simulink model "OFDM_Simulation_QPSK_rs1"  (R2018b)
settings: Solver=ode45  StartTime=0.0  StopTime=0.08  RelTol=1e-3  EnableMultiTasking=on
undefined symbols (not defined in the file or in its folder): doppler, rsgenpoly
libraries: dspindex x4, commdigbbndpm3 x4, commchan3 x2, commblkcod2 x2, commseqgen2 x2, commutil2 x2, dspxfrm3 x2, commrandsrc2 x1, commsink2 x1, dspobslib x1, dspsigops x1
settings Model: Creator=Three  LastModifiedBy=18831
settings SolverCC: MaxConsecutiveZCs=10
settings DataIOCC: LimitDataPoints=on  SaveFormat=Array
settings OptimizationCC: LifeSpan=inf
settings DebuggingCC: SolverPrmCheckMsg=warning  SFUnexpectedBacktrackingDiag=warning  SFNoUnconditionalDefaultTransitionDiag=warning  SFExecutionAtInitializationDiag=none
settings HardwareCC: ProdBitPerPointer=32  ProdBitPerSizeT=32  ProdBitPerPtrDiffT=32  ProdLargestAtomicFloat=None  ProdIntDivRoundTo=Undefined  ProdEndianess=Unspecified  ProdWordSize=32  ProdHWDeviceType=32-bit Generic
settings ModelReferenceCC: PropagateSignalLabelsOutOfModel=off
settings SFSimCC: SimUseLocalCustomCode=off
settings RTWCC: RTWUseLocalCustomCode=off
settings CodeAppCC: StateflowObjectComments=on
settings GRTTargetCC: TargetLangStandard=C89/C90 (ANSI)  GeneratePreprocessorConditionals=Disable all
settings ConfigComp: CovMetricSettings=dw  CovHtmlReporting=on  CovSaveCumulativeToWorkspaceVar=on  CovSaveSingleToWorkspaceVar=on  CovExternalEMLEnable=off  CovSFcnEnable=off

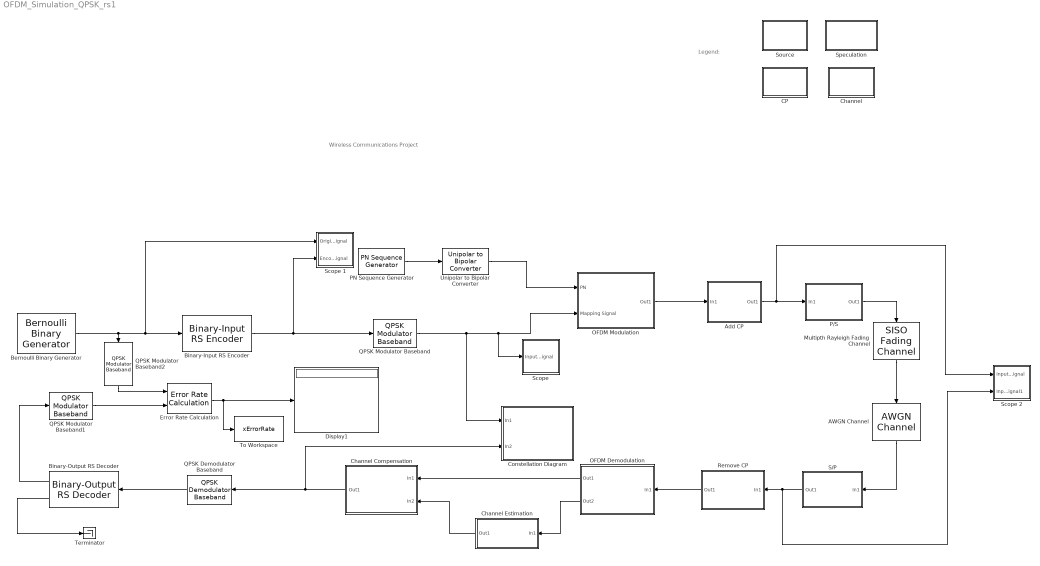
== system OFDM_Simulation_QPSK_rs1 ==
  note: Legend:
  note: Wireless Communications Project
  " Add CP" : Subsystem  TreatAsAtomicUnit=on
      mask Display: disp('Add CP')
  AWGN Channel : commchan3/AWGN Channel  InputProcessing=Columns as channels (frame based)  seed=17  noiseMode="Signal to noise ratio  (SNR)"  EbNodB=10  EsNodB=10  SNRdB=20  bitsPerSym=1  Ps=0.007  Tsym=1  variance=1
  Bernoulli Binary Generator : commrandsrc2/Bernoulli Binary Generator  P=0.5  seed=9044  Ts=16e-5/88/2  frameBased=on  sampPerFrame=88  orient=off  outDataType=double
  Binary-Input RS Encoder : commblkcod2/Binary-Input RS Encoder  n=15  k=11  specShortening=off  shortenedK=3  specGenPoly=off  genPoly=rsgenpoly(7,3)  specPrimPoly=off  prPoly=[1 0 1 1]  specPuncture=off  punctVec=[ones(2,1); zeros(2,1)]  outDType=Same as input
      settings: SourceProductName=Communications System Toolbox  SourceProductBaseCode=CM
  Binary-Output RS Decoder : commblkcod2/Binary-Output RS Decoder  n=15  k=11  specShortening=off  shortenedK=3  specGenPoly=off  genPoly=rsgenpoly(7,3)  specPrimPoly=off  prPoly=[1 0 1 1]  specPuncture=off  punctVec=[ones(2,1); zeros(2,1)]  specErasurePort=off  showNumErr=on  outDType=Same as input
      settings: SourceProductName=Communications System Toolbox  SourceProductBaseCode=CM
  CP : Subsystem  TreatAsAtomicUnit=on
      mask Display: disp('CP')
  Channel : Subsystem  TreatAsAtomicUnit=on
      mask Display: disp('Channel')
  Channel Compensation : Subsystem  TreatAsAtomicUnit=on
      mask Display: disp('Channel Compensation')
  Channel Estimation : Subsystem  TreatAsAtomicUnit=on
      mask Display: disp('Channel Estimation')
  Constellation Diagram : Subsystem  TreatAsAtomicUnit=on
      mask Display: disp('Constellation Diagram')
  Display1 : Display
  Error Rate Calculation : commsink2/Error Rate Calculation  N=44  st_delay=0  cp_mode=Entire frame  subframe=[]  PMode=Port  WsName=xErrorRate  RsMode2=off  stop=off  numErr=100  maxBits=1e6
  Multipth Rayleigh Fading Channel : commchan3/SISO Fading Channel  InheritSampleRate=on  SampleRate=1  PathDelays=[0 2e-6]  AveragePathGains=[0 -3]  NormalizePathGains=on  FadingDistribution=Rayleigh  KFactor=3  DirectPathDopplerShift=0  DirectPathInitialPhase=0  MaximumDopplerShift=100  DopplerSpectrum=doppler('Jakes')  ChannelInterpolationMethod=Polyphase  RandomStream=mt19937ar with seed  RandomNumGenerator=shr3cong  Seed=8007  PathGainsOutputPort=off  ChannelFilterDelayOutputPort=off  SimulateUsing=Interpreted execution  Visualization=Off  PathsForDopplerDisplay=1  SamplesToDisplay=25%
      settings: SourceProductName=Communications System Toolbox
  OFDM Demodulation : Subsystem  TreatAsAtomicUnit=on
      mask Display: disp('OFDM Demodulation')
  OFDM Modulation : Subsystem  TreatAsAtomicUnit=on
      mask Display: disp('OFDM Modulation')
  P/S : Subsystem  TreatAsAtomicUnit=on
      mask Display: disp('P/S')
  PN Sequence Generator : commseqgen2/PN Sequence Generator  poly=[1 0 0 0 0 1 1]  ini_sta=[0 0 0 0 0 1]  outBitMaskSource=Dialog parameter  shift=0  outVarSiz=off  maxOutSizeMode=Dialog parameter  maxOutSize=[10 1]  Ts=16e-5/2/61  frameBased=on  sampPerFrame=61  reset=off  bitPackedOutputs=off  outDataType=double  numPackedBits=8  bitPackDataSigned=off  bitPackedOutDType=double
  QPSK Demodulator Baseband : commdigbbndpm3/QPSK Demodulator Baseband  OutType=Bit  DecType=Hard decision  VarSource=Dialog  Variance=1  Dec=Gray  Ph=pi/4  outDtype1=Inherit via internal rule  outDtype2=Inherit via internal rule  derotateFactorWordLen=16  derotateFactorDataTypeStr=Inherit: Same word length as input  derotateFactorLastDataTypeStr=Inherit: Same word length as input
  QPSK Modulator Baseband : commdigbbndpm3/QPSK Modulator Baseband  InType=Bit  Enc=Gray  Ph=pi/4  outDtype=double  outWordLen=16  outUDDataType=sfix(16)  outFracLenMode=Best precision  outFracLen=15  outDataTypeStr=double  outLastDataTypeStr=double
  QPSK Modulator Baseband1 : commdigbbndpm3/QPSK Modulator Baseband  InType=Bit  Enc=Binary  Ph=pi/4  outDtype=double  outWordLen=16  outUDDataType=sfix(16)  outFracLenMode=Best precision  outFracLen=15  outDataTypeStr=double  outLastDataTypeStr=double
  QPSK Modulator Baseband2 : commdigbbndpm3/QPSK Modulator Baseband  InType=Bit  Enc=Binary  Ph=pi/4  outDtype=double  outWordLen=16  outUDDataType=sfix(16)  outFracLenMode=Best precision  outFracLen=15  outDataTypeStr=double  outLastDataTypeStr=double
  Remove CP : Subsystem  TreatAsAtomicUnit=on
      mask Display: disp('Remove CP')
  S/P : Subsystem  TreatAsAtomicUnit=on
      mask Display: disp('S/P')
  "Scope " : Subsystem
      mask Display: disp('Scope')
  Scope 1 : Subsystem
      mask Display: disp('Scope')
  Scope 2 : Subsystem
      mask Display: disp('Scope')
  Source : Subsystem  TreatAsAtomicUnit=on
      mask Display: disp('Source')
  Speculation : Subsystem  TreatAsAtomicUnit=on
      mask Display: disp('Speculation')
  Terminator : Terminator
  To Workspace : ToWorkspace  VariableName=xErrorRate  SampleTime=-1
      settings: Save2DSignal=2-D array (concatenate along first dimension)
  Unipolar to Bipolar Converter : commutil2/Unipolar to Bipolar Converter  M=2  polarity=Positive  dataType=Inherit via internal rule
      settings: SourceProductName=Communications System Toolbox
  wires:
  PN Sequence Generator/1 -> Unipolar to Bipolar Converter/1
  Unipolar to Bipolar Converter/1 -> OFDM Modulation/1(PN)
  QPSK Modulator Baseband/1 -> "Scope "/1(Input Signal), OFDM Modulation/2(Mapping Signal), Constellation Diagram/1(In1)
  Bernoulli Binary Generator/1 -> QPSK Modulator Baseband2/1, Scope 1/1(Original Signal), Binary-Input RS Encoder/1
  OFDM Modulation/1(Out1) -> " Add CP"/1(In1)
  " Add CP"/1(Out1) -> Scope 2/1(Input Signal), P/S/1(In1)
  AWGN Channel/1 -> S/P/1(In1)
  Remove CP/1(Out1) -> OFDM Demodulation/1(In1)
  OFDM Demodulation/2(Out2) -> Channel Estimation/1(In1)
  Channel Estimation/1(Out1) -> Channel Compensation/2(In2)
  OFDM Demodulation/1(Out1) -> Channel Compensation/1(In1)
  Channel Compensation/1(Out1) -> Constellation Diagram/2(In2), QPSK Demodulator Baseband/1
  QPSK Modulator Baseband1/1 -> Error Rate Calculation/2
  QPSK Modulator Baseband2/1 -> Error Rate Calculation/1
  P/S/1(Out1) -> Multipth Rayleigh Fading Channel/1
  Multipth Rayleigh Fading Channel/1 -> AWGN Channel/1
  Binary-Output RS Decoder/2 -> Terminator/1
  Binary-Input RS Encoder/1 -> QPSK Modulator Baseband/1, Scope 1/2(Encoded Signal)
  Error Rate Calculation/1 -> To Workspace/1, Display1/1
  QPSK Demodulator Baseband/1 -> Binary-Output RS Decoder/1
  Binary-Output RS Decoder/1 -> QPSK Modulator Baseband1/1
  S/P/1(Out1) -> Scope 2/2(Input Signal1), Remove CP/1(In1)

== system OFDM_Simulation_QPSK_rs1/ Add CP ==
  In1 : Inport
  Selector : Selector  NumberOfDimensions=2  InputPortWidth=3  IndexOptions=Index vector (dialog),Select all  Indices=[39:64,1:64],1  OutputSizes=1,1
  Out1 : Outport
  wires:
  In1/1 -> Selector/1
  Selector/1 -> Out1/1

== system OFDM_Simulation_QPSK_rs1/CP ==

== system OFDM_Simulation_QPSK_rs1/Channel ==

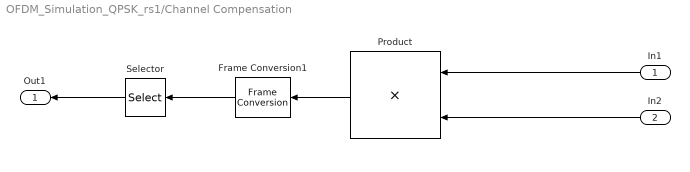
== system OFDM_Simulation_QPSK_rs1/Channel Compensation ==
  In1 : Inport
  In2 : Inport  Port=2
  Frame Conversion1 : FrameConversion
  Product : Product
  Selector : Selector  NumberOfDimensions=2  InputPortWidth=3  IndexOptions=Index vector (dialog),Select all  Indices=[1:30,32:61],1  OutputSizes=1,1
  Out1 : Outport
  wires:
  In1/1 -> Product/1
  In2/1 -> Product/2
  Product/1 -> Frame Conversion1/1
  Frame Conversion1/1 -> Selector/1
  Selector/1 -> Out1/1

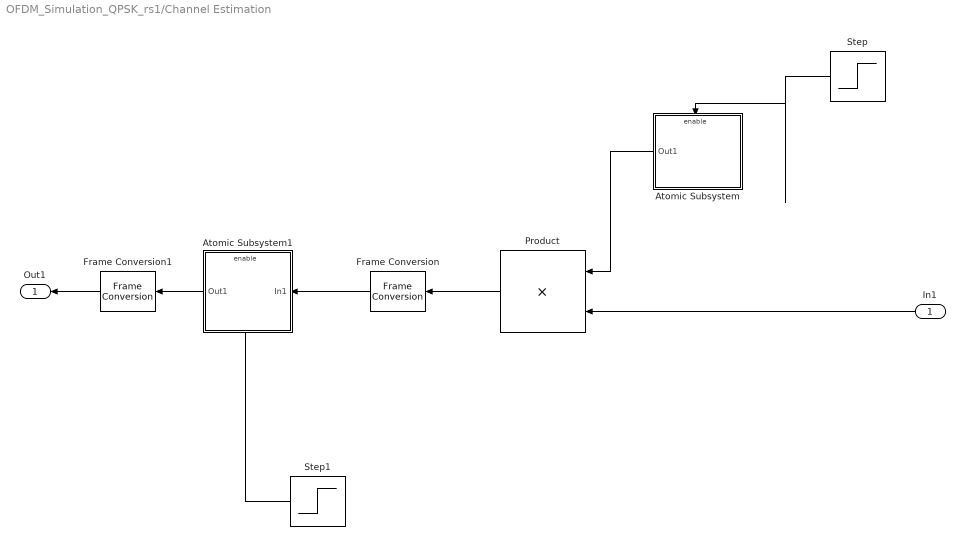
== system OFDM_Simulation_QPSK_rs1/Channel Estimation ==
  In1 : Inport
  Atomic Subsystem : Subsystem  TreatAsAtomicUnit=on
  Atomic Subsystem1 : Subsystem  TreatAsAtomicUnit=on
  Frame Conversion : FrameConversion
  Frame Conversion1 : FrameConversion
  Product : Product
  Step : Step  Time=16e-5/2  SampleTime=0
  Step1 : Step  Time=16e-5/2  SampleTime=0
  Out1 : Outport
  wires:
  In1/1 -> Product/2
  Step/1 -> Atomic Subsystem/Enable
  Atomic Subsystem/1(Out1) -> Product/1
  Product/1 -> Frame Conversion/1
  Frame Conversion/1 -> Atomic Subsystem1/1(In1)
  Step1/1 -> Atomic Subsystem1/Enable
  Atomic Subsystem1/1(Out1) -> Frame Conversion1/1
  Frame Conversion1/1 -> Out1/1

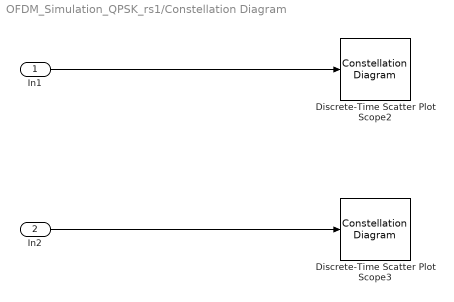
== system OFDM_Simulation_QPSK_rs1/Constellation Diagram ==
  In1 : Inport
  In2 : Inport  Port=2
  Discrete-Time Scatter Plot Scope2 : ConstellationDiagram  Tag=ScatterPlot
  Discrete-Time Scatter Plot Scope3 : ConstellationDiagram  Tag=ScatterPlot
  wires:
  In2/1 -> Discrete-Time Scatter Plot Scope3/1
  In1/1 -> Discrete-Time Scatter Plot Scope2/1

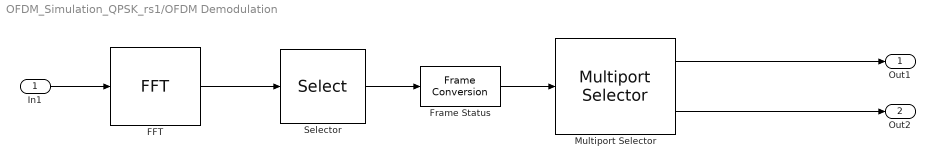
== system OFDM_Simulation_QPSK_rs1/OFDM Demodulation ==
  In1 : Inport
  FFT : dspxfrm3/FFT  FFTImplementation=Auto  CompMethod=Table lookup  TableOpt=NEW  TableOptActive=Speed  BitRevOrder=off  Normalize=off  InheritFFTLength=on  FFTLength=64  WrapInput=on  roundingMode=Floor  overflowMode=off  firstCoeffDataTypeStr=Inherit: Same word length as input  firstCoeffLastDataTypeStr=Inherit: Same word length as input  outputMin=[]  outputMax=[]
  Frame Status : FrameConversion
  Multiport Selector : dspindex/Multiport Selector  rowsOrCols=Columns  idxCellArray={1,2}  idxErrMode=Clip Index
  Selector : Selector  NumberOfDimensions=2  InputPortWidth=3  IndexOptions=Index vector (dialog),Select all  Indices=[35:64,1:31],1  OutputSizes=1,1
  Out1 : Outport
  Out2 : Outport  Port=2
  wires:
  In1/1 -> FFT/1
  FFT/1 -> Selector/1
  Selector/1 -> Frame Status/1
  Frame Status/1 -> Multiport Selector/1
  Multiport Selector/2 -> Out2/1
  Multiport Selector/1 -> Out1/1

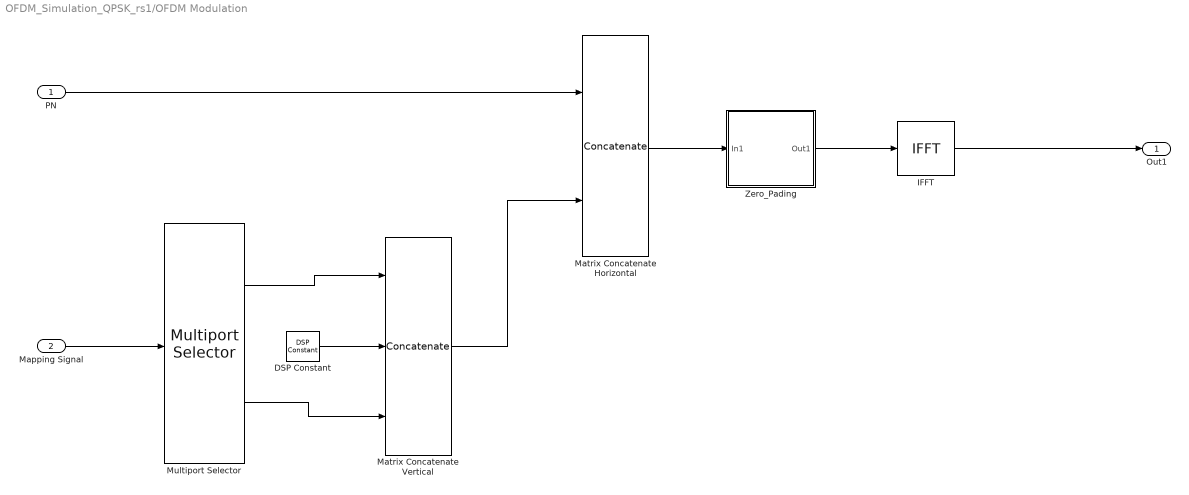
== system OFDM_Simulation_QPSK_rs1/OFDM Modulation ==
  PN : Inport
  Mapping Signal : Inport  Port=2
  DSP Constant : dspobslib/DSP Constant  Value=0  SampleMode=Discrete  discreteOutput=Frame-based  continuousOutput=Sample-based  sampTime=16e-5/2  framePeriod=16e-5/2  dataType=Inherit from 'Constant value'  isSigned=on  wordLen=16  udDataType=sfix(16)  fracBitsMode=Best precision  numFracBits=15  InterpretAs1D=off  Ts=16e-5/2  FramebasedOutput=on
      settings: SourceProductName=DSP System Toolbox  SourceProductBaseCode=DS
  IFFT : dspxfrm3/IFFT  FFTImplementation=Auto  CompMethod=Table lookup  TableOpt=NEW  TableOptActive=Speed  BitRevOrder=off  cs_in=off  Normalize=on  InheritFFTLength=on  FFTLength=64  WrapInput=on  mode=Complex  outSamplingMode=Frame based  roundingMode=Floor  overflowMode=off  firstCoeffDataTypeStr=Inherit: Same word length as input  firstCoeffLastDataTypeStr=Inherit: Same word length as input  outputMin=[]  outputMax=[]
      settings: SourceProductName=DSP System Toolbox
  Matrix Concatenate Horizontal : Concatenate  Mode=Multidimensional array  ConcatenateDimension=2
  Matrix Concatenate Vertical : Concatenate  NumInputs=3  Mode=Multidimensional array
  Multiport Selector : dspindex/Multiport Selector  rowsOrCols=Rows  idxCellArray={1:30,31:60}  idxErrMode=Clip Index
  Zero_Pading : Subsystem  TreatAsAtomicUnit=on
      mask Display: disp('Zero_Pading')
  Out1 : Outport
  wires:
  Mapping Signal/1 -> Multiport Selector/1
  PN/1 -> Matrix Concatenate Horizontal/1
  Multiport Selector/1 -> Matrix Concatenate Vertical/1
  Multiport Selector/2 -> Matrix Concatenate Vertical/3
  DSP Constant/1 -> Matrix Concatenate Vertical/2
  Matrix Concatenate Vertical/1 -> Matrix Concatenate Horizontal/2
  Matrix Concatenate Horizontal/1 -> Zero_Pading/1(In1)
  Zero_Pading/1(Out1) -> IFFT/1
  IFFT/1 -> Out1/1

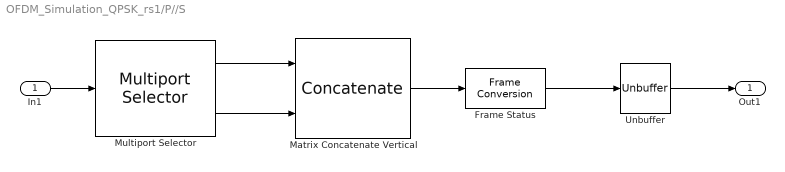
== system OFDM_Simulation_QPSK_rs1/P//S ==
  In1 : Inport
  Frame Status : FrameConversion
  Matrix Concatenate Vertical : Concatenate  Mode=Multidimensional array
  Multiport Selector : dspindex/Multiport Selector  rowsOrCols=Columns  idxCellArray={1,2}  idxErrMode=Clip Index
  Unbuffer : Unbuffer
  Out1 : Outport
  wires:
  In1/1 -> Multiport Selector/1
  Multiport Selector/1 -> Matrix Concatenate Vertical/1
  Multiport Selector/2 -> Matrix Concatenate Vertical/2
  Matrix Concatenate Vertical/1 -> Frame Status/1
  Frame Status/1 -> Unbuffer/1
  Unbuffer/1 -> Out1/1

== system OFDM_Simulation_QPSK_rs1/Remove CP ==
  In1 : Inport
  Selector : Selector  NumberOfDimensions=2  InputPortWidth=3  IndexOptions=Index vector (dialog),Select all  Indices=[27:90],1  OutputSizes=1,1
  Out1 : Outport
  wires:
  In1/1 -> Selector/1
  Selector/1 -> Out1/1

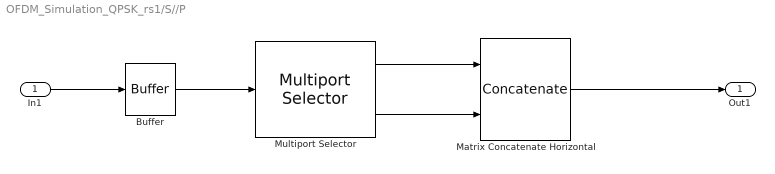
== system OFDM_Simulation_QPSK_rs1/S//P ==
  In1 : Inport
  Buffer : Buffer  N=180
  Matrix Concatenate Horizontal : Concatenate  Mode=Multidimensional array  ConcatenateDimension=2
  Multiport Selector : dspindex/Multiport Selector  rowsOrCols=Rows  idxCellArray={91:180,1:90}  idxErrMode=Clip Index
  Out1 : Outport
  wires:
  In1/1 -> Buffer/1
  Buffer/1 -> Multiport Selector/1
  Multiport Selector/1 -> Matrix Concatenate Horizontal/1
  Multiport Selector/2 -> Matrix Concatenate Horizontal/2
  Matrix Concatenate Horizontal/1 -> Out1/1

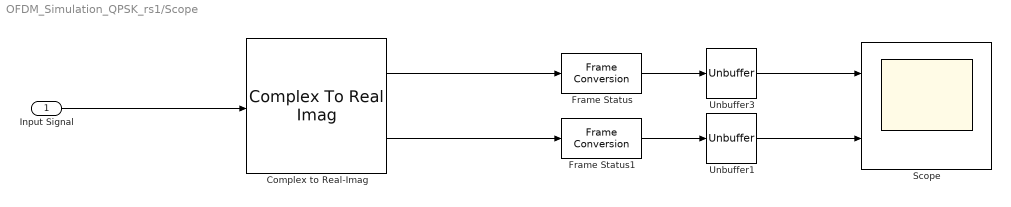
== system OFDM_Simulation_QPSK_rs1/Scope  ==
  Input Signal : Inport
  Complex to Real-Imag : ComplexToRealImag
  Frame Status : FrameConversion  OutFrame=Sample-based
  Frame Status1 : FrameConversion  OutFrame=Sample-based
  Scope : Scope  NumInputPorts=2
  Unbuffer1 : Unbuffer
  Unbuffer3 : Unbuffer
  wires:
  Input Signal/1 -> Complex to Real-Imag/1
  Complex to Real-Imag/2 -> Frame Status1/1
  Frame Status1/1 -> Unbuffer1/1
  Unbuffer1/1 -> Scope/2
  Unbuffer3/1 -> Scope/1
  Complex to Real-Imag/1 -> Frame Status/1
  Frame Status/1 -> Unbuffer3/1

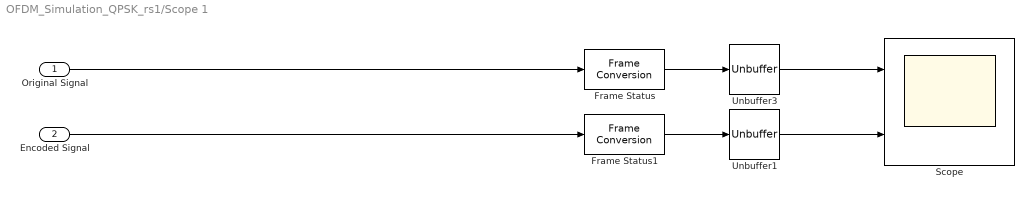
== system OFDM_Simulation_QPSK_rs1/Scope 1 ==
  Original Signal : Inport
  Encoded Signal : Inport  Port=2
  Frame Status : FrameConversion  OutFrame=Sample-based
  Frame Status1 : FrameConversion  OutFrame=Sample-based
  Scope : Scope  NumInputPorts=2
  Unbuffer1 : Unbuffer
  Unbuffer3 : Unbuffer
  wires:
  Frame Status1/1 -> Unbuffer1/1
  Unbuffer1/1 -> Scope/2
  Unbuffer3/1 -> Scope/1
  Frame Status/1 -> Unbuffer3/1
  Encoded Signal/1 -> Frame Status1/1
  Original Signal/1 -> Frame Status/1

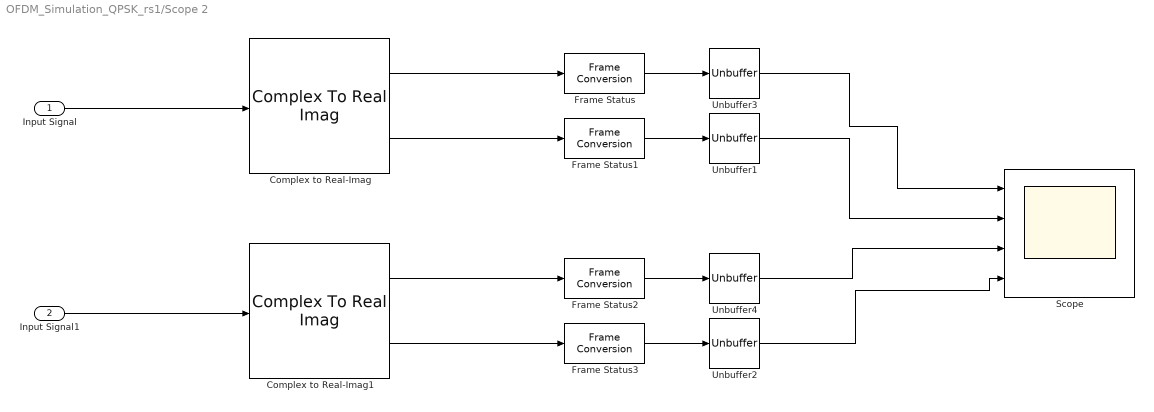
== system OFDM_Simulation_QPSK_rs1/Scope 2 ==
  Input Signal : Inport
  Input Signal1 : Inport  Port=2
  Complex to Real-Imag : ComplexToRealImag
  Complex to Real-Imag1 : ComplexToRealImag
  Frame Status{,1..3} (4 alike) : FrameConversion  OutFrame=Sample-based
  Scope : Scope  NumInputPorts=4
  Unbuffer{1..4} (4 alike) : Unbuffer
  wires:
  Input Signal/1 -> Complex to Real-Imag/1
  Complex to Real-Imag/2 -> Frame Status1/1
  Frame Status1/1 -> Unbuffer1/1
  Unbuffer1/1 -> Scope/2
  Unbuffer3/1 -> Scope/1
  Complex to Real-Imag/1 -> Frame Status/1
  Frame Status/1 -> Unbuffer3/1
  Input Signal1/1 -> Complex to Real-Imag1/1
  Complex to Real-Imag1/2 -> Frame Status3/1
  Frame Status3/1 -> Unbuffer2/1
  Unbuffer2/1 -> Scope/4
  Unbuffer4/1 -> Scope/3
  Complex to Real-Imag1/1 -> Frame Status2/1
  Frame Status2/1 -> Unbuffer4/1

== system OFDM_Simulation_QPSK_rs1/Source ==

== system OFDM_Simulation_QPSK_rs1/Speculation ==

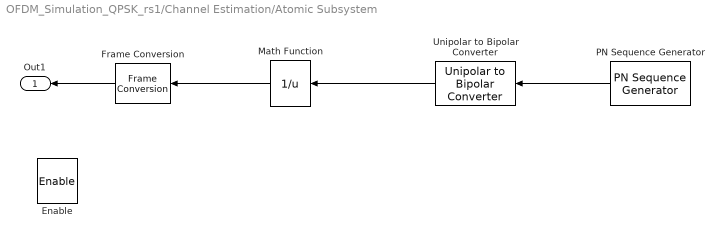
== system OFDM_Simulation_QPSK_rs1/Channel Estimation/Atomic Subsystem ==
  Enable : EnablePort
  Frame Conversion : FrameConversion
  Math Function : Math  Operator=reciprocal  SaturateOnIntegerOverflow=on
  PN Sequence Generator : commseqgen2/PN Sequence Generator  poly=[1 0 0 0 0 1 1]  ini_sta=[0 0 0 0 0 1]  outBitMaskSource=Dialog parameter  shift=0  outVarSiz=off  maxOutSizeMode=Dialog parameter  maxOutSize=[10 1]  Ts=16e-5/2/61  frameBased=on  sampPerFrame=61  reset=off  bitPackedOutputs=off  outDataType=double  numPackedBits=8  bitPackDataSigned=off  bitPackedOutDType=double
  Unipolar to Bipolar Converter : commutil2/Unipolar to Bipolar Converter  M=2  polarity=Positive  dataType=Inherit via internal rule
      settings: SourceProductName=Communications System Toolbox
  Out1 : Outport
  wires:
  PN Sequence Generator/1 -> Unipolar to Bipolar Converter/1
  Frame Conversion/1 -> Out1/1
  Unipolar to Bipolar Converter/1 -> Math Function/1
  Math Function/1 -> Frame Conversion/1

== system OFDM_Simulation_QPSK_rs1/Channel Estimation/Atomic Subsystem1 ==
  In1 : Inport
  Enable : EnablePort
  Math Function : Math  Operator=reciprocal  SaturateOnIntegerOverflow=on
  Out1 : Outport
  wires:
  In1/1 -> Math Function/1
  Math Function/1 -> Out1/1

== system OFDM_Simulation_QPSK_rs1/OFDM Modulation/Zero_Pading ==
  In1 : Inport
  Pad : dspsigops/Pad  padAlong=Columns and rows  dimsToPad=1  valSrc=Specify via dialog  padVal=0  spec=Output size  padNumOutRowsSpecMethod=User-specified  numOutRows=64  padNumOutColsSpecMethod=User-specified  numOutCols=2  isVarDimsMode=off  padBeginning=0  padEnd=0  outSizeMode=User-specified  outSize=1  padSigAt=End  trunc_flag=None  roundingMode=Floor  overflowMode=off  truncOrWrapMode=Truncate  wrap_flag=None
      settings: SourceProductName=DSP System Toolbox  SourceProductBaseCode=DS
  Selector : Selector  NumberOfDimensions=2  InputPortWidth=3  IndexOptions=Index vector (dialog),Select all  Indices=[31:64,1:30],1  OutputSizes=1,1
  Out1 : Outport
  wires:
  In1/1 -> Pad/1
  Pad/1 -> Selector/1
  Selector/1 -> Out1/1
